simulink model "sampleModel1838"  (R2023a)
settings: Solver=VariableStepAuto  StartTime=0.0  StopTime=10.0  RelTol=1e-3
libraries: hdlsllib x5
settings Model: Creator=user1  LastModifiedBy=user1

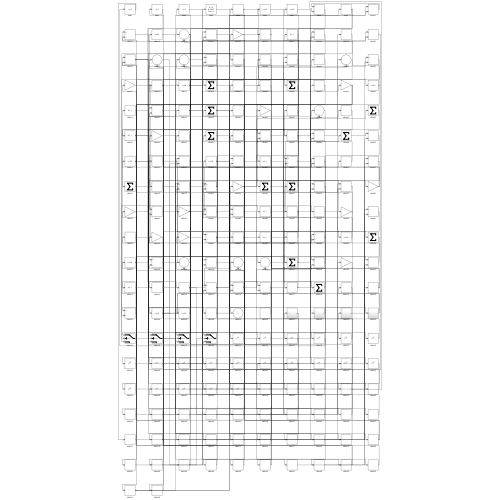
[thumbnail: Simulink's stored preview of the top-level diagram]
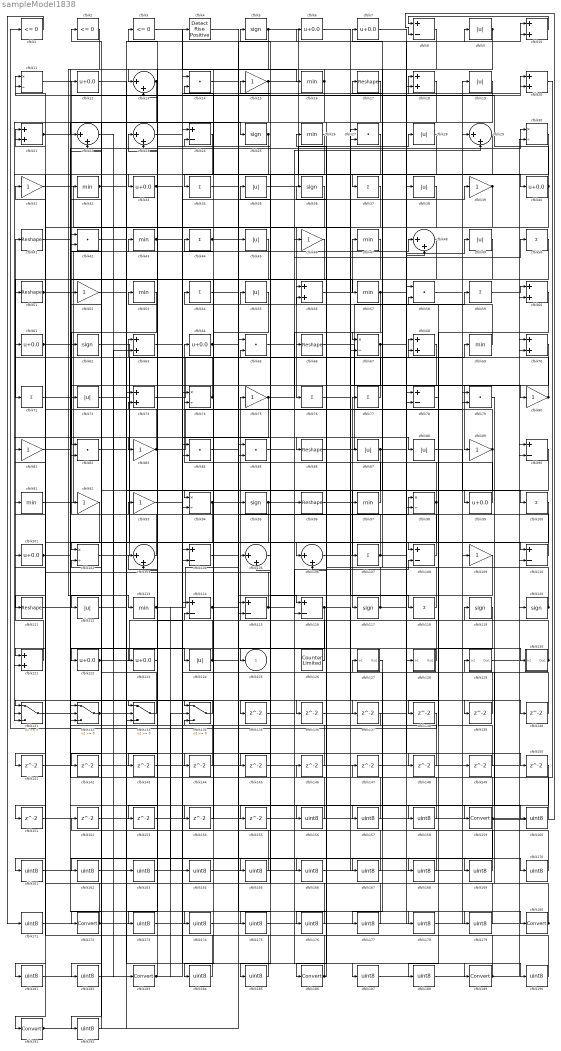
== system sampleModel1838 ==
  cfblk1 : hdlsllib/Logic and Bit Operations/Compare To Zero  relop=<=  OutDataTypeStr=boolean
  cfblk{10,18,20..21,56,60,63,68,70,73,121} (11 alike) : Sum
  cfblk{34,37,44,50,54,59,71,76..77,100,107,118} (12 alike) : Sum  Inputs=+
  cfblk{6..7,12,33,40,61,64,99,101,122..123} (11 alike) : Bias  Bias=0.0  SaturateOnIntegerOverflow=off
  cfblk{11,30,67,74,94,98,102} (7 alike) : Product  Inputs=*/  RndMeth=Zero  SaturateOnIntegerOverflow=on
  cfblk{13,22..23,29,48,103,105..106} (8 alike) : Sum  Inputs=|++
  cfblk{8,24,78,90,104,108,110,114..116} (10 alike) : Sum  Inputs=+-
  cfblk{15,31,39,46,52,75,80..81,83,89,92..93,109} (13 alike) : Gain
  cfblk{17,41,51,66,86,96,111} (7 alike) : Reshape
  cfblk{9,19,28,35,38,45,49,55,72,87..88,112,124} (13 alike) : Abs  SaturateOnIntegerOverflow=off
  cfblk{16,26,32,43,47,53,57,69,91,97,113} (11 alike) : MinMax
  cfblk{5,25,36,62,95,117,119..120} (8 alike) : Signum
  cfblk126 : hdlsllib/Sources/Counter Limited  uplimit=7  tsamp=-1
  cfblk127 : Subsystem
      settings: LibrarySourceBlock=|
      | hdlsllib/Ports &
      | Subsystems/Subsystem
  cfblk128 : Subsystem
      settings: LibrarySourceBlock=|
      | hdlsllib/Ports &
      | Subsystems/Subsystem
  cfblk129 : Subsystem
      settings: LibrarySourceBlock=|
      | hdlsllib/Ports &
      | Subsystems/Subsystem
  cfblk130 : Subsystem
      settings: LibrarySourceBlock=|
      | hdlsllib/Ports &
      | Subsystems/Subsystem
  cfblk{131..134} (4 alike) : Switch  SaturateOnIntegerOverflow=off  InputSameDT=off
  cfblk{135..155} (21 alike) : Delay  SampleTime=1
  cfblk{14,27,42,58,65,79,82,84..85} (9 alike) : DotProduct  OutDataTypeStr=Inherit: Inherit via internal rule
  cfblk{156..158,160..171,173..179,181..182,184..185,187..188,190,192} (30 alike) : DataTypeConversion  OutDataTypeStr=uint8  SaturateOnIntegerOverflow=off  RndMeth=Floor
  cfblk{159,172,180,183,186,189,191} (7 alike) : DataTypeConversion  SaturateOnIntegerOverflow=off  RndMeth=Floor
  cfblk2 : hdlsllib/Logic and Bit Operations/Compare To Zero  relop=<=  OutDataTypeStr=boolean
  cfblk3 : hdlsllib/Logic and Bit Operations/Compare To Zero  relop=<=  OutDataTypeStr=boolean
  cfblk4 : hdlsllib/Logic and Bit Operations/Detect Rise Positive  vinit=0  OutDataTypeStr=boolean
  cfblk125 : Outport  VectorParamsAs1DForOutWhenUnconnected=off
  wires:
  cfblk108/1 -> cfblk12/1
  cfblk132/1 -> cfblk140/1, cfblk174/1
  cfblk78/1 -> cfblk102/1
  cfblk79/1 -> cfblk159/1
  cfblk2/1 -> cfblk113/1
  cfblk55/1 -> cfblk134/1
  cfblk126/1 -> cfblk75/1
  cfblk77/1 -> cfblk3/1
  cfblk23/1 -> cfblk18/1
  cfblk72/1 -> cfblk110/1
  cfblk96/1 -> cfblk117/1
  cfblk91/1 -> cfblk43/1
  cfblk59/1 -> cfblk60/1
  cfblk56/1 -> cfblk47/1
  cfblk99/1 -> cfblk64/1
  cfblk104/1 -> cfblk98/1
  cfblk102/1 -> cfblk68/1
  cfblk103/1 -> cfblk93/1
  cfblk121/1 -> cfblk41/1
  cfblk35/1 -> cfblk28/1
  cfblk70/1 -> cfblk172/1
  cfblk113/1 -> cfblk69/1, cfblk164/1
  cfblk97/1 -> cfblk55/1
  cfblk92/1 -> cfblk191/1
  cfblk86/1 -> cfblk59/1
  cfblk67/1 -> cfblk49/1, cfblk82/2
  cfblk94/1 -> cfblk157/1, cfblk161/1
  cfblk46/1 -> cfblk112/1
  cfblk18/1 -> cfblk67/1
  cfblk53/1 -> cfblk82/1
  cfblk123/1 -> cfblk103/1
  cfblk62/1 -> cfblk99/1
  cfblk111/1 -> cfblk48/1
  cfblk50/1 -> cfblk76/1
  cfblk17/1 -> cfblk72/1
  cfblk110/1 -> cfblk44/1
  cfblk116/1 -> cfblk132/2, cfblk139/1
  cfblk118/1 -> cfblk7/1
  cfblk29/1 -> cfblk111/1
  cfblk16/1 -> cfblk13/1, cfblk143/1
  cfblk120/1 -> cfblk54/1, cfblk63/1
  cfblk73/1 -> cfblk38/1
  cfblk106/1 -> cfblk77/1
  cfblk9/1 -> cfblk97/1, cfblk123/1
  cfblk6/1 -> cfblk118/1
  cfblk66/1 -> cfblk89/1
  cfblk30/1 -> cfblk33/1
  cfblk22/1 -> cfblk183/1
  cfblk130/1(Out1) -> cfblk119/1, cfblk114/2
  cfblk64/1 -> cfblk130/1(In1), cfblk137/1
  cfblk80/1 -> cfblk68/2, cfblk32/1
  cfblk39/1 -> cfblk66/1, cfblk145/1, cfblk181/1
  cfblk101/1 -> cfblk30/1, cfblk21/1
  cfblk131/1 -> cfblk62/1
  cfblk14/1 -> cfblk88/1
  cfblk32/1 -> cfblk94/1, cfblk122/1
  cfblk43/1 -> cfblk39/1, cfblk86/1
  cfblk88/1 -> cfblk100/1
  cfblk89/1 -> cfblk31/1, cfblk106/1
  cfblk8/1 -> cfblk34/1
  cfblk44/1 -> cfblk116/1, cfblk57/1
  cfblk34/1 -> cfblk95/1
  cfblk122/1 -> cfblk4/1, cfblk74/1, cfblk63/2
  cfblk90/1 -> cfblk186/1
  cfblk69/1 -> cfblk5/1
  cfblk75/1 -> cfblk46/1, cfblk29/2, cfblk131/2
  cfblk21/1 -> cfblk25/1, cfblk154/1, cfblk168/1
  cfblk84/1 -> cfblk180/1
  cfblk31/1 -> cfblk87/1
  cfblk33/1 -> cfblk37/1, cfblk190/1
  cfblk25/1 -> cfblk131/3, cfblk153/1
  cfblk117/1 -> cfblk48/2, cfblk26/1
  cfblk51/1 -> cfblk56/1, cfblk136/1
  cfblk48/1 -> cfblk71/1
  cfblk40/1 -> cfblk121/1, cfblk11/2
  cfblk5/1 -> cfblk40/1, cfblk132/3
  cfblk124/1 -> cfblk53/1, cfblk6/1
  cfblk83/1 -> cfblk104/2, cfblk29/1, cfblk73/2
  cfblk54/1 -> cfblk115/1
  cfblk60/1 -> cfblk108/1
  cfblk74/1 -> cfblk2/1, cfblk11/1
  cfblk128/1(Out1) -> cfblk35/1
  cfblk133/1 -> cfblk102/2
  cfblk52/1 -> cfblk189/1
  cfblk63/1 -> cfblk20/1
  cfblk15/1 -> cfblk128/1(In1), cfblk133/2
  cfblk134/1 -> cfblk131/1
  cfblk11/1 -> cfblk20/2
  cfblk58/1 -> cfblk19/1
  cfblk24/1 -> cfblk83/1
  cfblk57/1 -> cfblk116/2, cfblk10/2
  cfblk114/1 -> cfblk65/1, cfblk10/1
  cfblk112/1 -> cfblk9/1
  cfblk61/1 -> cfblk124/1, cfblk148/1
  cfblk115/1 -> cfblk108/2, cfblk91/1
  cfblk107/1 -> cfblk78/1, cfblk74/2
  cfblk68/1 -> cfblk125/1
  cfblk76/1 -> cfblk80/1
  cfblk71/1 -> cfblk107/1
  cfblk36/1 -> cfblk51/1
  cfblk129/1(Out1) -> cfblk60/2
  cfblk65/1 -> cfblk50/1
  cfblk98/1 -> cfblk17/1, cfblk106/2
  cfblk10/1 -> cfblk8/1
  cfblk3/1 -> cfblk16/1
  cfblk87/1 -> cfblk78/2, cfblk142/1
  cfblk13/1 -> cfblk121/2, cfblk133/1
  cfblk95/1 -> cfblk96/1, cfblk182/1
  cfblk37/1 -> cfblk135/1
  cfblk136/1 -> cfblk18/2
  cfblk137/1 -> cfblk134/3
  cfblk119/1 -> cfblk138/1
  cfblk138/1 -> cfblk1/1
  cfblk139/1 -> cfblk24/2
  cfblk140/1 -> cfblk104/1
  cfblk38/1 -> cfblk141/1
  cfblk141/1 -> cfblk94/2
  cfblk142/1 -> cfblk98/2
  cfblk143/1 -> cfblk114/1
  cfblk41/1 -> cfblk144/1
  cfblk144/1 -> cfblk132/1
  cfblk145/1 -> cfblk110/2
  cfblk146/1 -> cfblk23/2
  cfblk20/1 -> cfblk147/1
  cfblk148/1 -> cfblk65/2
  cfblk149/1 -> cfblk58/2
  cfblk7/1 -> cfblk150/1
  cfblk45/1 -> cfblk151/1
  cfblk151/1 -> cfblk30/2
  cfblk153/1 -> cfblk67/2
  cfblk154/1 -> cfblk14/2
  cfblk28/1 -> cfblk155/1
  cfblk155/1 -> cfblk15/1
  cfblk42/1 -> cfblk156/1
  cfblk156/1 -> cfblk103/2
  cfblk157/1 -> cfblk42/1
  cfblk4/1 -> cfblk158/1
  cfblk158/1 -> cfblk42/2
  cfblk159/1 -> cfblk8/2, cfblk24/1, cfblk192/1
  cfblk93/1 -> cfblk160/1
  cfblk160/1 -> cfblk79/1
  cfblk161/1 -> cfblk79/2
  cfblk27/1 -> cfblk162/1
  cfblk162/1 -> cfblk73/1
  cfblk12/1 -> cfblk163/1
  cfblk163/1 -> cfblk27/1
  cfblk164/1 -> cfblk27/2
  cfblk109/1 -> cfblk165/1
  cfblk165/1 -> cfblk14/1
  cfblk19/1 -> cfblk166/1
  cfblk166/1 -> cfblk109/1
  cfblk127/1(Out1) -> cfblk167/1
  cfblk167/1 -> cfblk152/1
  cfblk168/1 -> cfblk127/1(In1)
  cfblk85/1 -> cfblk169/1
  cfblk169/1 -> cfblk23/1
  cfblk152/1 -> cfblk170/1
  cfblk170/1 -> cfblk85/1
  cfblk1/1 -> cfblk171/1
  cfblk171/1 -> cfblk85/2
  cfblk172/1 -> cfblk61/1, cfblk120/1
  cfblk26/1 -> cfblk173/1
  cfblk173/1 -> cfblk70/1
  cfblk174/1 -> cfblk70/2
  cfblk105/1 -> cfblk175/1
  cfblk175/1 -> cfblk58/1
  cfblk49/1 -> cfblk176/1
  cfblk176/1 -> cfblk105/1
  cfblk147/1 -> cfblk177/1
  cfblk177/1 -> cfblk105/2
  cfblk81/1 -> cfblk178/1
  cfblk178/1 -> cfblk149/1
  cfblk82/1 -> cfblk179/1
  cfblk179/1 -> cfblk81/1
  cfblk180/1 -> cfblk146/1, cfblk129/1(In1)
  cfblk181/1 -> cfblk84/1
  cfblk182/1 -> cfblk84/2
  cfblk183/1 -> cfblk13/2, cfblk134/2
  cfblk47/1 -> cfblk184/1
  cfblk184/1 -> cfblk22/1
  cfblk150/1 -> cfblk185/1
  cfblk185/1 -> cfblk22/2
  cfblk186/1 -> cfblk56/2, cfblk101/1
  cfblk135/1 -> cfblk187/1
  cfblk187/1 -> cfblk90/1
  cfblk100/1 -> cfblk188/1
  cfblk188/1 -> cfblk90/2
  cfblk189/1 -> cfblk21/2, cfblk36/1
  cfblk190/1 -> cfblk52/1
  cfblk191/1 -> cfblk133/3, cfblk115/2, cfblk45/1
  cfblk192/1 -> cfblk92/1

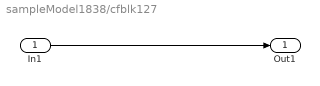
== system sampleModel1838/cfblk127 ==
  In1 : Inport
  Out1 : Outport
  wires:
  In1/1 -> Out1/1

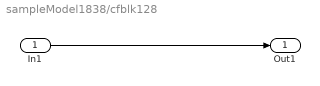
== system sampleModel1838/cfblk128 ==
  In1 : Inport
  Out1 : Outport
  wires:
  In1/1 -> Out1/1

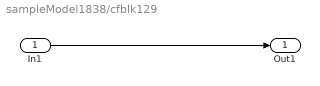
== system sampleModel1838/cfblk129 ==
  In1 : Inport
  Out1 : Outport
  wires:
  In1/1 -> Out1/1

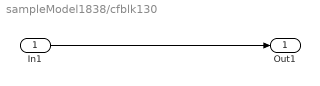
== system sampleModel1838/cfblk130 ==
  In1 : Inport
  Out1 : Outport
  wires:
  In1/1 -> Out1/1
